simulink model "flockingModel"  (R2018b)
settings: Solver=FixedStepAuto  StartTime=0.0  StopTime=300  FixedStep=0.01  RelTol=1e-3
values from neighbouring files (symbols this model uses):
  a = 0.15    [diff_drive.m]    (also in main.m)
  bias = 0.2    [diff_drive.m]    (also in main.m)
  obsR = 0.15    [main.m]
  theta01 = 0    [main.m]
  theta02 = pi/2    (= 1.57079632679)    [main.m]
  theta03 = pi/4    (= 0.785398163397)    [main.m]
  w = 0.1    [diff_drive.m]    (also in main.m)
  x01 = 0.2    [main.m]
  x02 = 0.07    [main.m]
  x03 = 0.05    [main.m]
  x_obs = 0.20    (= 0.2)    [diff_drive.m]    (also in main.m = 1.5)
  x_star = 0.15    [diff_drive.m]    (also in main.m = 2.2)
  y01 = 0.25    [main.m]
  y02 = 0.5    [main.m]
  y03 = 0.3    [main.m]
  y_obs = 0.2    [diff_drive.m]    (also in main.m = 1)
  y_star = 0.00    (= 0)    [diff_drive.m]    (also in main.m = 1)
settings Model: Creator=root  LastModifiedBy=root

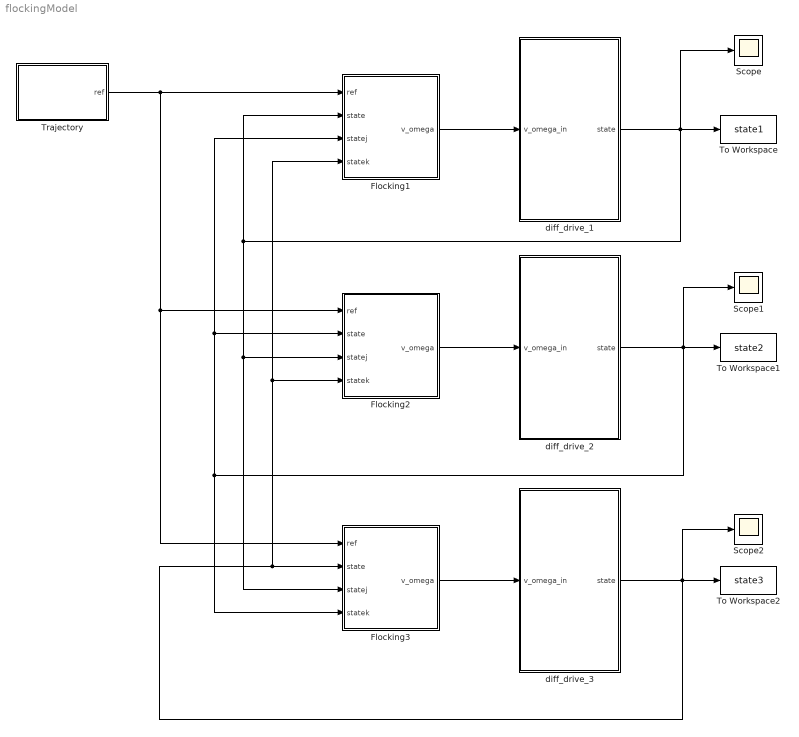
== system flockingModel ==
  Flocking1 : Subsystem
  Flocking2 : Subsystem
  Flocking3 : Subsystem
  Scope : Scope
  Scope1 : Scope
  Scope2 : Scope
  To Workspace : ToWorkspace  VariableName=state1  SaveFormat=Timeseries  SampleTime=-1
  To Workspace1 : ToWorkspace  VariableName=state2  SaveFormat=Timeseries  SampleTime=-1
  To Workspace2 : ToWorkspace  VariableName=state3  SaveFormat=Timeseries  SampleTime=-1
  Trajectory : Subsystem  TreatAsAtomicUnit=on
  diff_drive_1 : Subsystem  mask{base=0.078, base_error=2.5, radius=0.029, radius_error=6.9, omega_max=180}
      mask prompts: base_error "Base error in percent"; radius_error "Radius error in percent"; omega_max "Wheel Max Velocity"
  "diff_drive_2 " : Subsystem  mask{base=0.078, base_error=2.5, radius=0.029, radius_error=6.9, omega_max=180}
      mask prompts: base_error "Base error in percent"; radius_error "Radius error in percent"; omega_max "Wheel Max Velocity"
  diff_drive_3 : Subsystem  mask{base=0.078, base_error=2.5, radius=0.029, radius_error=6.9, omega_max=180}
      mask prompts: base_error "Base error in percent"; radius_error "Radius error in percent"; omega_max "Wheel Max Velocity"
  wires:
  Trajectory/1(ref) -> Flocking1/1(ref), Flocking3/1(ref), Flocking2/1(ref)
  diff_drive_1/1(state) -> Scope/1, To Workspace/1, Flocking1/2(state), Flocking3/3(statej), Flocking2/3(statej)
  Flocking1/1(v_omega) -> diff_drive_1/1(v_omega_in)
  "diff_drive_2 "/1(state) -> Scope1/1, To Workspace1/1, Flocking3/4(statek), Flocking2/2(state), Flocking1/3(statej)
  Flocking2/1(v_omega) -> "diff_drive_2 "/1(v_omega_in)
  Flocking3/1(v_omega) -> diff_drive_3/1(v_omega_in)
  diff_drive_3/1(state) -> Scope2/1, Flocking3/2(state), Flocking2/4(statek), Flocking1/4(statek), To Workspace2/1

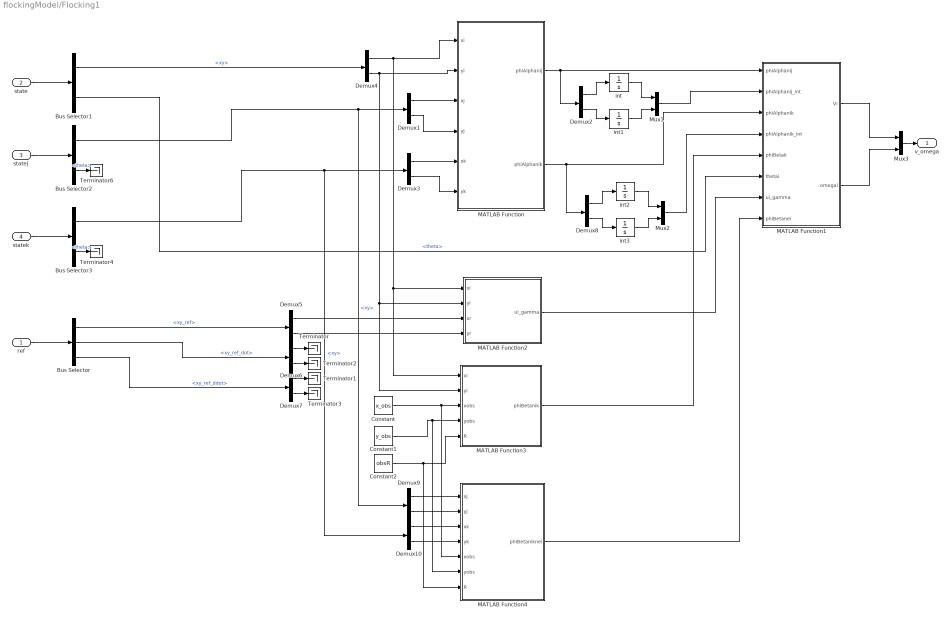
== system flockingModel/Flocking1 ==
  ref : Inport
  state : Inport  Port=2
  statej : Inport  Port=3
  statek : Inport  Port=4
  Bus Selector : BusSelector  OutputSignals=xy_ref,xy_ref_dot,xy_ref_ddot
  Bus Selector1 : BusSelector  OutputSignals=xy,theta
  Bus Selector2 : BusSelector  OutputSignals=xy,theta
  Bus Selector3 : BusSelector  OutputSignals=xy,theta
  Constant : Constant  Value=x_obs
  Constant1 : Constant  Value=y_obs
  Constant2 : Constant  Value=obsR
  Demux{1..10} (10 alike) : Demux  Outputs=2
  MATLAB Function : MATLAB Function  TreatAsAtomicUnit=on
  MATLAB Function1 : MATLAB Function  TreatAsAtomicUnit=on
  MATLAB Function2 : MATLAB Function  TreatAsAtomicUnit=on
  MATLAB Function3 : MATLAB Function  TreatAsAtomicUnit=on
  MATLAB Function4 : MATLAB Function  TreatAsAtomicUnit=on
  Mux1 : Mux  Inputs=2
  Mux2 : Mux  Inputs=2
  Mux3 : Mux  Inputs=2
  Terminator{,1..4,6} (6 alike) : Terminator
  int{,1..3} (4 alike) : Integrator
  v_omega : Outport
  wires:
  ref/1 -> Bus Selector/1
  state/1 -> Bus Selector1/1
  Bus Selector/2 -> Demux6/1  "<xy_ref_dot>"
  Bus Selector/1 -> Demux5/1  "<xy_ref>"
  Bus Selector/3 -> Demux7/1  "<xy_ref_ddot>"
  Bus Selector1/1 -> Demux4/1  "<xy>"
  Mux3/1 -> v_omega/1
  Demux6/1 -> Terminator/1
  Demux6/2 -> Terminator2/1
  Demux7/1 -> Terminator1/1
  Demux7/2 -> Terminator3/1
  statej/1 -> Bus Selector2/1
  Bus Selector2/1 -> Demux9/1, Demux1/1  "<xy>"
  Demux4/1 -> MATLAB Function/1(xi), MATLAB Function3/1(xi), MATLAB Function2/1(xi)
  Demux4/2 -> MATLAB Function/2(yi), MATLAB Function3/2(yi), MATLAB Function2/2(yi)
  Demux1/1 -> MATLAB Function/3(xj)
  Demux1/2 -> MATLAB Function/4(yj)
  MATLAB Function1/1(Vi) -> Mux3/1
  MATLAB Function1/2(omegai) -> Mux3/2
  MATLAB Function/1(phiAlphanij) -> Demux2/1, MATLAB Function1/1(phiAlphanij)
  Demux5/2 -> MATLAB Function2/4(yr)
  Bus Selector2/2 -> Terminator6/1  "<theta>"
  Bus Selector1/2 -> MATLAB Function1/6(thetai)  "<theta>"
  Demux2/1 -> int/1
  Demux2/2 -> int1/1
  int/1 -> Mux1/1
  int1/1 -> Mux1/2
  Mux1/1 -> MATLAB Function1/2(phiAlphanij_int)
  Demux5/1 -> MATLAB Function2/3(xr)
  MATLAB Function2/1(ui_gamma) -> MATLAB Function1/7(ui_gamma)
  statek/1 -> Bus Selector3/1
  Bus Selector3/2 -> Terminator4/1  "<theta>"
  Demux3/1 -> MATLAB Function/5(xk)
  Demux3/2 -> MATLAB Function/6(yk)
  Bus Selector3/1 -> Demux10/1, Demux3/1  "<xy>"
  int3/1 -> Mux2/2
  MATLAB Function/2(phiAlphanik) -> Demux8/1, MATLAB Function1/3(phiAlphanik)
  Demux8/1 -> int2/1
  Demux8/2 -> int3/1
  int2/1 -> Mux2/1
  Mux2/1 -> MATLAB Function1/4(phiAlphanik_int)
  Constant/1 -> MATLAB Function4/5(xobs), MATLAB Function3/3(xobs)
  Constant1/1 -> MATLAB Function4/6(yobs), MATLAB Function3/4(yobs)
  MATLAB Function3/1(phiBetanik) -> MATLAB Function1/5(phiBetak)
  Constant2/1 -> MATLAB Function4/7(R), MATLAB Function3/5(R)
  Demux9/1 -> MATLAB Function4/1(xj)
  Demux9/2 -> MATLAB Function4/2(yj)
  Demux10/1 -> MATLAB Function4/3(xk)
  Demux10/2 -> MATLAB Function4/4(yk)
  MATLAB Function4/1(phiBetaniknei) -> MATLAB Function1/8(phiBetanei)

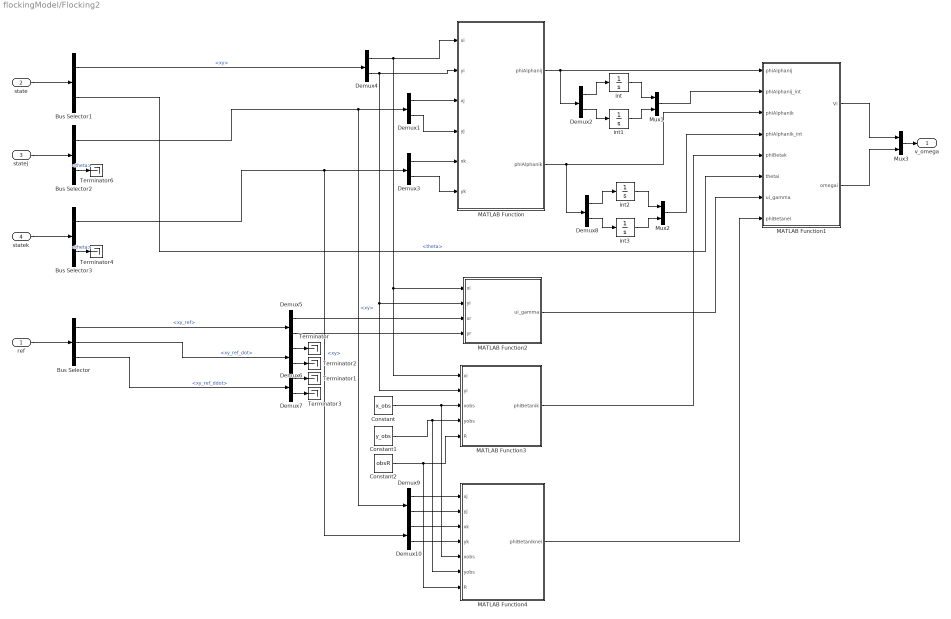
== system flockingModel/Flocking2 ==
  ref : Inport
  state : Inport  Port=2
  statej : Inport  Port=3
  statek : Inport  Port=4
  Bus Selector : BusSelector  OutputSignals=xy_ref,xy_ref_dot,xy_ref_ddot
  Bus Selector1 : BusSelector  OutputSignals=xy,theta
  Bus Selector2 : BusSelector  OutputSignals=xy,theta
  Bus Selector3 : BusSelector  OutputSignals=xy,theta
  Constant : Constant  Value=x_obs
  Constant1 : Constant  Value=y_obs
  Constant2 : Constant  Value=obsR
  Demux{1..10} (10 alike) : Demux  Outputs=2
  MATLAB Function : MATLAB Function  TreatAsAtomicUnit=on
  MATLAB Function1 : MATLAB Function  TreatAsAtomicUnit=on
  MATLAB Function2 : MATLAB Function  TreatAsAtomicUnit=on
  MATLAB Function3 : MATLAB Function  TreatAsAtomicUnit=on
  MATLAB Function4 : MATLAB Function  TreatAsAtomicUnit=on
  Mux1 : Mux  Inputs=2
  Mux2 : Mux  Inputs=2
  Mux3 : Mux  Inputs=2
  Terminator{,1..4,6} (6 alike) : Terminator
  int{,1..3} (4 alike) : Integrator
  v_omega : Outport
  wires:
  ref/1 -> Bus Selector/1
  state/1 -> Bus Selector1/1
  Bus Selector/2 -> Demux6/1  "<xy_ref_dot>"
  Bus Selector/1 -> Demux5/1  "<xy_ref>"
  Bus Selector/3 -> Demux7/1  "<xy_ref_ddot>"
  Bus Selector1/1 -> Demux4/1  "<xy>"
  Mux3/1 -> v_omega/1
  Demux6/1 -> Terminator/1
  Demux6/2 -> Terminator2/1
  Demux7/1 -> Terminator1/1
  Demux7/2 -> Terminator3/1
  statej/1 -> Bus Selector2/1
  Bus Selector2/1 -> Demux9/1, Demux1/1  "<xy>"
  Demux4/1 -> MATLAB Function/1(xi), MATLAB Function3/1(xi), MATLAB Function2/1(xi)
  Demux4/2 -> MATLAB Function/2(yi), MATLAB Function3/2(yi), MATLAB Function2/2(yi)
  Demux1/1 -> MATLAB Function/3(xj)
  Demux1/2 -> MATLAB Function/4(yj)
  MATLAB Function1/1(Vi) -> Mux3/1
  MATLAB Function1/2(omegai) -> Mux3/2
  MATLAB Function/1(phiAlphanij) -> Demux2/1, MATLAB Function1/1(phiAlphanij)
  Demux5/2 -> MATLAB Function2/4(yr)
  Bus Selector2/2 -> Terminator6/1  "<theta>"
  Bus Selector1/2 -> MATLAB Function1/6(thetai)  "<theta>"
  Demux2/1 -> int/1
  Demux2/2 -> int1/1
  int/1 -> Mux1/1
  int1/1 -> Mux1/2
  Mux1/1 -> MATLAB Function1/2(phiAlphanij_int)
  Demux5/1 -> MATLAB Function2/3(xr)
  MATLAB Function2/1(ui_gamma) -> MATLAB Function1/7(ui_gamma)
  statek/1 -> Bus Selector3/1
  Bus Selector3/2 -> Terminator4/1  "<theta>"
  Demux3/1 -> MATLAB Function/5(xk)
  Demux3/2 -> MATLAB Function/6(yk)
  Bus Selector3/1 -> Demux10/1, Demux3/1  "<xy>"
  int3/1 -> Mux2/2
  MATLAB Function/2(phiAlphanik) -> Demux8/1, MATLAB Function1/3(phiAlphanik)
  Demux8/1 -> int2/1
  Demux8/2 -> int3/1
  int2/1 -> Mux2/1
  Mux2/1 -> MATLAB Function1/4(phiAlphanik_int)
  Constant/1 -> MATLAB Function4/5(xobs), MATLAB Function3/3(xobs)
  Constant1/1 -> MATLAB Function4/6(yobs), MATLAB Function3/4(yobs)
  MATLAB Function3/1(phiBetanik) -> MATLAB Function1/5(phiBetak)
  Constant2/1 -> MATLAB Function4/7(R), MATLAB Function3/5(R)
  Demux9/1 -> MATLAB Function4/1(xj)
  Demux9/2 -> MATLAB Function4/2(yj)
  Demux10/1 -> MATLAB Function4/3(xk)
  Demux10/2 -> MATLAB Function4/4(yk)
  MATLAB Function4/1(phiBetaniknei) -> MATLAB Function1/8(phiBetanei)

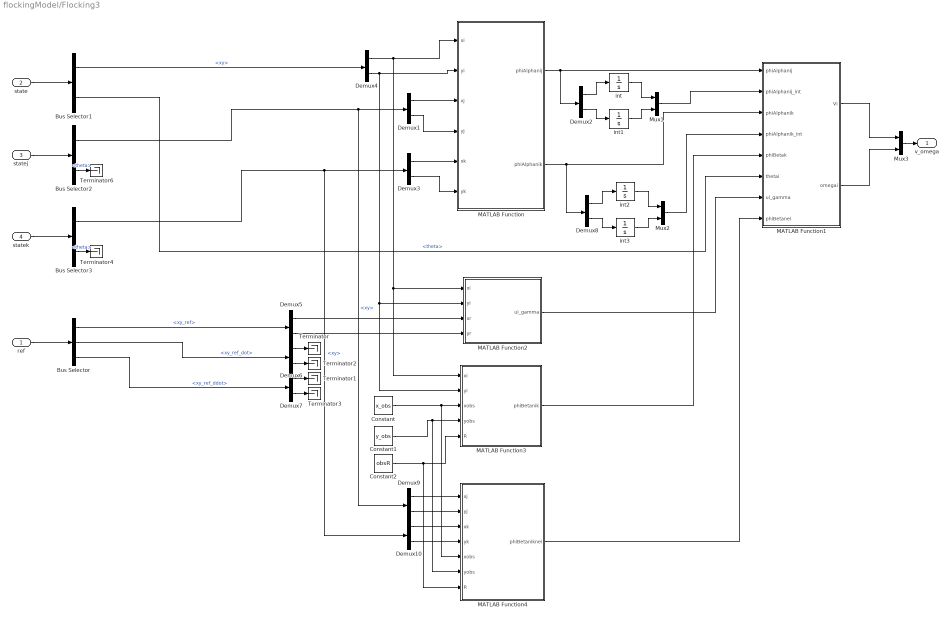
== system flockingModel/Flocking3 ==
  ref : Inport
  state : Inport  Port=2
  statej : Inport  Port=3
  statek : Inport  Port=4
  Bus Selector : BusSelector  OutputSignals=xy_ref,xy_ref_dot,xy_ref_ddot
  Bus Selector1 : BusSelector  OutputSignals=xy,theta
  Bus Selector2 : BusSelector  OutputSignals=xy,theta
  Bus Selector3 : BusSelector  OutputSignals=xy,theta
  Constant : Constant  Value=x_obs
  Constant1 : Constant  Value=y_obs
  Constant2 : Constant  Value=obsR
  Demux{1..10} (10 alike) : Demux  Outputs=2
  MATLAB Function : MATLAB Function  TreatAsAtomicUnit=on
  MATLAB Function1 : MATLAB Function  TreatAsAtomicUnit=on
  MATLAB Function2 : MATLAB Function  TreatAsAtomicUnit=on
  MATLAB Function3 : MATLAB Function  TreatAsAtomicUnit=on
  MATLAB Function4 : MATLAB Function  TreatAsAtomicUnit=on
  Mux1 : Mux  Inputs=2
  Mux2 : Mux  Inputs=2
  Mux3 : Mux  Inputs=2
  Terminator{,1..4,6} (6 alike) : Terminator
  int{,1..3} (4 alike) : Integrator
  v_omega : Outport
  wires:
  ref/1 -> Bus Selector/1
  state/1 -> Bus Selector1/1
  Bus Selector/2 -> Demux6/1  "<xy_ref_dot>"
  Bus Selector/1 -> Demux5/1  "<xy_ref>"
  Bus Selector/3 -> Demux7/1  "<xy_ref_ddot>"
  Bus Selector1/1 -> Demux4/1  "<xy>"
  Mux3/1 -> v_omega/1
  Demux6/1 -> Terminator/1
  Demux6/2 -> Terminator2/1
  Demux7/1 -> Terminator1/1
  Demux7/2 -> Terminator3/1
  statej/1 -> Bus Selector2/1
  Bus Selector2/1 -> Demux9/1, Demux1/1  "<xy>"
  Demux4/1 -> MATLAB Function/1(xi), MATLAB Function3/1(xi), MATLAB Function2/1(xi)
  Demux4/2 -> MATLAB Function/2(yi), MATLAB Function3/2(yi), MATLAB Function2/2(yi)
  Demux1/1 -> MATLAB Function/3(xj)
  Demux1/2 -> MATLAB Function/4(yj)
  MATLAB Function1/1(Vi) -> Mux3/1
  MATLAB Function1/2(omegai) -> Mux3/2
  MATLAB Function/1(phiAlphanij) -> Demux2/1, MATLAB Function1/1(phiAlphanij)
  Demux5/2 -> MATLAB Function2/4(yr)
  Bus Selector2/2 -> Terminator6/1  "<theta>"
  Bus Selector1/2 -> MATLAB Function1/6(thetai)  "<theta>"
  Demux2/1 -> int/1
  Demux2/2 -> int1/1
  int/1 -> Mux1/1
  int1/1 -> Mux1/2
  Mux1/1 -> MATLAB Function1/2(phiAlphanij_int)
  Demux5/1 -> MATLAB Function2/3(xr)
  MATLAB Function2/1(ui_gamma) -> MATLAB Function1/7(ui_gamma)
  statek/1 -> Bus Selector3/1
  Bus Selector3/2 -> Terminator4/1  "<theta>"
  Demux3/1 -> MATLAB Function/5(xk)
  Demux3/2 -> MATLAB Function/6(yk)
  Bus Selector3/1 -> Demux10/1, Demux3/1  "<xy>"
  int3/1 -> Mux2/2
  MATLAB Function/2(phiAlphanik) -> Demux8/1, MATLAB Function1/3(phiAlphanik)
  Demux8/1 -> int2/1
  Demux8/2 -> int3/1
  int2/1 -> Mux2/1
  Mux2/1 -> MATLAB Function1/4(phiAlphanik_int)
  Constant/1 -> MATLAB Function4/5(xobs), MATLAB Function3/3(xobs)
  Constant1/1 -> MATLAB Function4/6(yobs), MATLAB Function3/4(yobs)
  MATLAB Function3/1(phiBetanik) -> MATLAB Function1/5(phiBetak)
  Constant2/1 -> MATLAB Function4/7(R), MATLAB Function3/5(R)
  Demux9/1 -> MATLAB Function4/1(xj)
  Demux9/2 -> MATLAB Function4/2(yj)
  Demux10/1 -> MATLAB Function4/3(xk)
  Demux10/2 -> MATLAB Function4/4(yk)
  MATLAB Function4/1(phiBetaniknei) -> MATLAB Function1/8(phiBetanei)

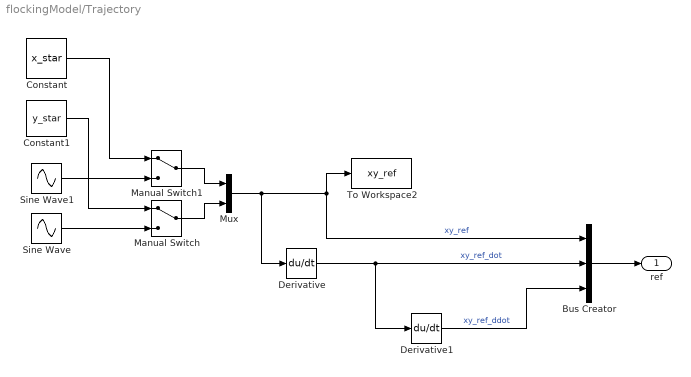
== system flockingModel/Trajectory ==
  Bus Creator : BusCreator  Inputs=3
  Constant : Constant  Value=x_star
  Constant1 : Constant  Value=y_star
  Derivative : Derivative
  Derivative1 : Derivative
  Manual Switch : ManualSwitch
  Manual Switch1 : ManualSwitch
  Mux : Mux  Inputs=2
  Sine Wave : Sin  Amplitude=a  Bias=bias  Frequency=w  SampleTime=0
  Sine Wave1 : Sin  Amplitude=a  Bias=bias  Frequency=w  Phase=pi/2  SampleTime=0
  To Workspace2 : ToWorkspace  VariableName=xy_ref  SampleTime=-1
      settings: Save2DSignal=2-D array (concatenate along first dimension)
  ref : Outport
  wires:
  Bus Creator/1 -> ref/1
  Mux/1 -> Derivative/1, Bus Creator/1, To Workspace2/1  "xy_ref"
  Derivative/1 -> Bus Creator/2, Derivative1/1  "xy_ref_dot"
  Derivative1/1 -> Bus Creator/3  "xy_ref_ddot"
  Sine Wave/1 -> Manual Switch/2
  Sine Wave1/1 -> Manual Switch1/2
  Constant/1 -> Manual Switch1/1
  Constant1/1 -> Manual Switch/1
  Manual Switch1/1 -> Mux/1
  Manual Switch/1 -> Mux/2

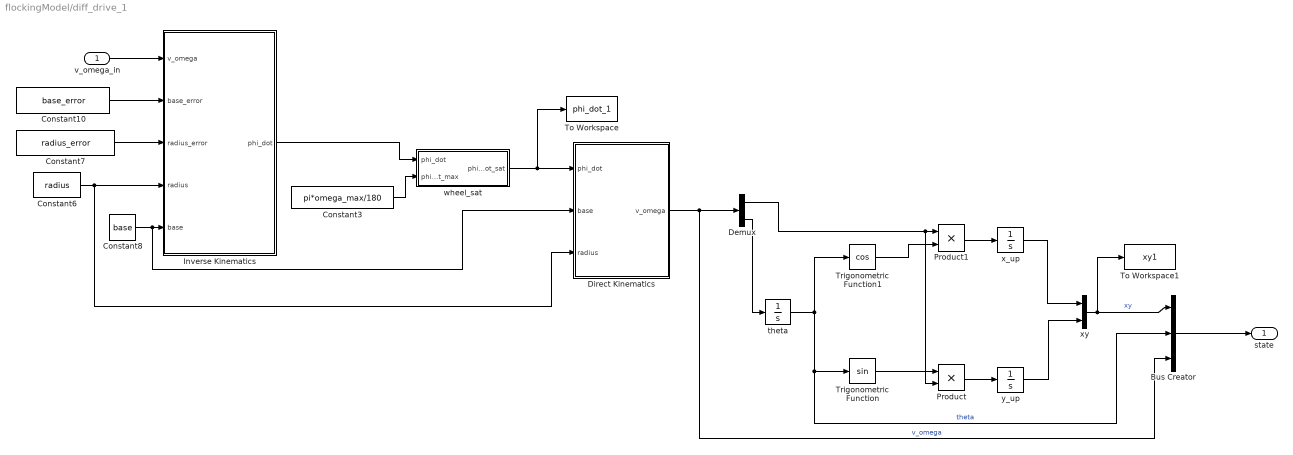
== system flockingModel/diff_drive_1 ==
  v_omega_in : Inport
  Bus Creator : BusCreator  Inputs=3
  Constant10 : Constant  Value=base_error
  Constant3 : Constant  Value=pi*omega_max/180
  Constant6 : Constant  Value=radius
  Constant7 : Constant  Value=radius_error
  Constant8 : Constant  Value=base
  Demux : Demux  Outputs=2
  Direct Kinematics : MATLAB Function  TreatAsAtomicUnit=on
  Inverse Kinematics : MATLAB Function  TreatAsAtomicUnit=on
  Product : Product
  Product1 : Product
  To Workspace : ToWorkspace  VariableName=phi_dot_1  SampleTime=-1
      settings: Save2DSignal=2-D array (concatenate along first dimension)
  To Workspace1 : ToWorkspace  VariableName=xy1  SampleTime=-1
      settings: Save2DSignal=2-D array (concatenate along first dimension)
  Trigonometric Function : Trigonometry
  Trigonometric Function1 : Trigonometry  Operator=cos
  theta : Integrator  InitialCondition=theta01
  wheel_sat : Subsystem
  x_up : Integrator  InitialCondition=x01
  xy : Mux  Inputs=2
  y_up : Integrator  InitialCondition=y01
  state : Outport
  wires:
  theta/1 -> Trigonometric Function1/1, Trigonometric Function/1, Bus Creator/2  "theta"
  Trigonometric Function1/1 -> Product1/2
  Trigonometric Function/1 -> Product/1
  Product/1 -> y_up/1
  Product1/1 -> x_up/1
  x_up/1 -> xy/1
  Constant3/1 -> wheel_sat/2(phi_dot_max)
  Direct Kinematics/1(v_omega) -> Bus Creator/3, Demux/1  "v_omega"
  Demux/1 -> Product/2, Product1/1
  Demux/2 -> theta/1
  y_up/1 -> xy/2
  wheel_sat/1(phi_dot_sat) -> Direct Kinematics/1(phi_dot), To Workspace/1
  xy/1 -> Bus Creator/1, To Workspace1/1  "xy"
  Bus Creator/1 -> state/1
  Inverse Kinematics/1(phi_dot) -> wheel_sat/1(phi_dot)
  v_omega_in/1 -> Inverse Kinematics/1(v_omega)
  Constant10/1 -> Inverse Kinematics/2(base_error)
  Constant7/1 -> Inverse Kinematics/3(radius_error)
  Constant6/1 -> Inverse Kinematics/4(radius), Direct Kinematics/3(radius)
  Constant8/1 -> Direct Kinematics/2(base), Inverse Kinematics/5(base)

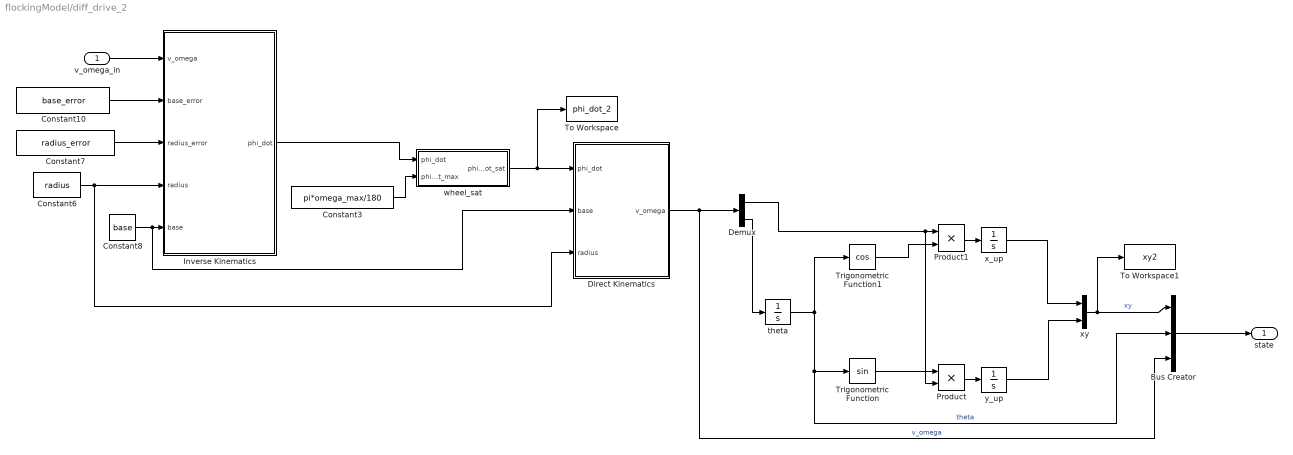
== system flockingModel/diff_drive_2  ==
  v_omega_in : Inport
  Bus Creator : BusCreator  Inputs=3
  Constant10 : Constant  Value=base_error
  Constant3 : Constant  Value=pi*omega_max/180
  Constant6 : Constant  Value=radius
  Constant7 : Constant  Value=radius_error
  Constant8 : Constant  Value=base
  Demux : Demux  Outputs=2
  Direct Kinematics : MATLAB Function  TreatAsAtomicUnit=on
  Inverse Kinematics : MATLAB Function  TreatAsAtomicUnit=on
  Product : Product
  Product1 : Product
  To Workspace : ToWorkspace  VariableName=phi_dot_2  SampleTime=-1
      settings: Save2DSignal=2-D array (concatenate along first dimension)
  To Workspace1 : ToWorkspace  VariableName=xy2  SampleTime=-1
      settings: Save2DSignal=2-D array (concatenate along first dimension)
  Trigonometric Function : Trigonometry
  Trigonometric Function1 : Trigonometry  Operator=cos
  theta : Integrator  InitialCondition=theta02
  wheel_sat : Subsystem
  x_up : Integrator  InitialCondition=x02
  xy : Mux  Inputs=2
  y_up : Integrator  InitialCondition=y02
  state : Outport
  wires:
  Constant8/1 -> Inverse Kinematics/5(base), Direct Kinematics/2(base)
  Constant6/1 -> Direct Kinematics/3(radius), Inverse Kinematics/4(radius)
  Constant7/1 -> Inverse Kinematics/3(radius_error)
  Constant10/1 -> Inverse Kinematics/2(base_error)
  v_omega_in/1 -> Inverse Kinematics/1(v_omega)
  Inverse Kinematics/1(phi_dot) -> wheel_sat/1(phi_dot)
  Bus Creator/1 -> state/1
  xy/1 -> To Workspace1/1, Bus Creator/1  "xy"
  wheel_sat/1(phi_dot_sat) -> To Workspace/1, Direct Kinematics/1(phi_dot)
  y_up/1 -> xy/2
  Demux/2 -> theta/1
  Demux/1 -> Product1/1, Product/2
  Direct Kinematics/1(v_omega) -> Demux/1, Bus Creator/3  "v_omega"
  Constant3/1 -> wheel_sat/2(phi_dot_max)
  x_up/1 -> xy/1
  Product1/1 -> x_up/1
  Product/1 -> y_up/1
  Trigonometric Function/1 -> Product/1
  Trigonometric Function1/1 -> Product1/2
  theta/1 -> Bus Creator/2, Trigonometric Function/1, Trigonometric Function1/1  "theta"

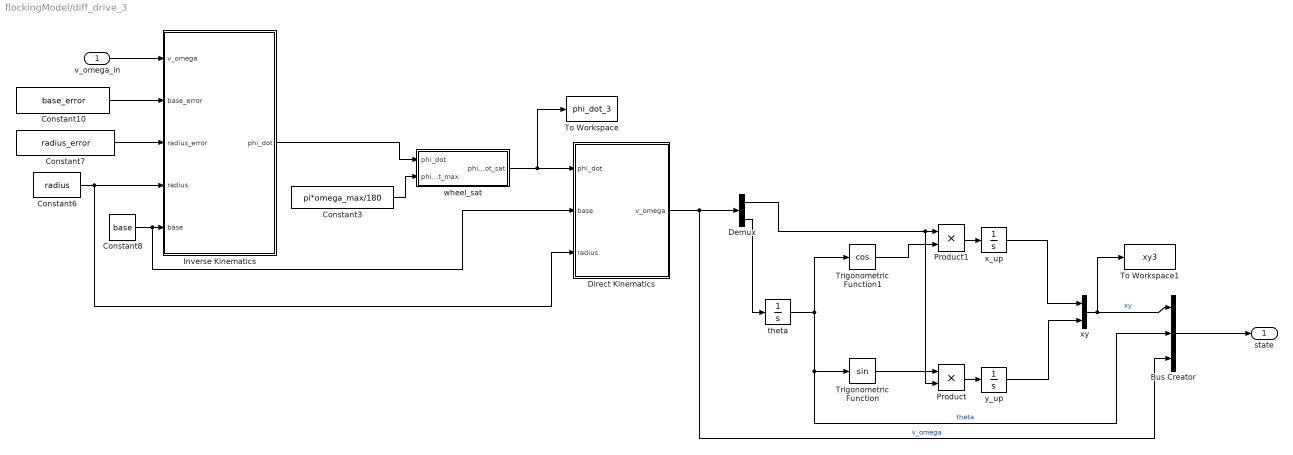
== system flockingModel/diff_drive_3 ==
  v_omega_in : Inport
  Bus Creator : BusCreator  Inputs=3
  Constant10 : Constant  Value=base_error
  Constant3 : Constant  Value=pi*omega_max/180
  Constant6 : Constant  Value=radius
  Constant7 : Constant  Value=radius_error
  Constant8 : Constant  Value=base
  Demux : Demux  Outputs=2
  Direct Kinematics : MATLAB Function  TreatAsAtomicUnit=on
  Inverse Kinematics : MATLAB Function  TreatAsAtomicUnit=on
  Product : Product
  Product1 : Product
  To Workspace : ToWorkspace  VariableName=phi_dot_3  SampleTime=-1
      settings: Save2DSignal=2-D array (concatenate along first dimension)
  To Workspace1 : ToWorkspace  VariableName=xy3  SampleTime=-1
      settings: Save2DSignal=2-D array (concatenate along first dimension)
  Trigonometric Function : Trigonometry
  Trigonometric Function1 : Trigonometry  Operator=cos
  theta : Integrator  InitialCondition=theta03
  wheel_sat : Subsystem
  x_up : Integrator  InitialCondition=x03
  xy : Mux  Inputs=2
  y_up : Integrator  InitialCondition=y03
  state : Outport
  wires:
  Constant8/1 -> Inverse Kinematics/5(base), Direct Kinematics/2(base)
  Constant6/1 -> Direct Kinematics/3(radius), Inverse Kinematics/4(radius)
  Constant7/1 -> Inverse Kinematics/3(radius_error)
  Constant10/1 -> Inverse Kinematics/2(base_error)
  v_omega_in/1 -> Inverse Kinematics/1(v_omega)
  Inverse Kinematics/1(phi_dot) -> wheel_sat/1(phi_dot)
  Bus Creator/1 -> state/1
  xy/1 -> To Workspace1/1, Bus Creator/1  "xy"
  wheel_sat/1(phi_dot_sat) -> To Workspace/1, Direct Kinematics/1(phi_dot)
  y_up/1 -> xy/2
  Demux/2 -> theta/1
  Demux/1 -> Product1/1, Product/2
  Direct Kinematics/1(v_omega) -> Demux/1, Bus Creator/3  "v_omega"
  Constant3/1 -> wheel_sat/2(phi_dot_max)
  x_up/1 -> xy/1
  Product1/1 -> x_up/1
  Product/1 -> y_up/1
  Trigonometric Function/1 -> Product/1
  Trigonometric Function1/1 -> Product1/2
  theta/1 -> Bus Creator/2, Trigonometric Function/1, Trigonometric Function1/1  "theta"

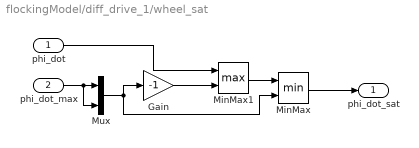
== system flockingModel/diff_drive_1/wheel_sat ==
  phi_dot : Inport
  phi_dot_max : Inport  Port=2
  Gain : Gain  Gain=-1
  MinMax : MinMax  Inputs=2
  MinMax1 : MinMax  Function=max  Inputs=2
  Mux : Mux  Inputs=2
  phi_dot_sat : Outport
  wires:
  Gain/1 -> MinMax1/2
  MinMax/1 -> phi_dot_sat/1
  phi_dot_max/1 -> Mux/2, Mux/1
  phi_dot/1 -> MinMax1/1
  MinMax1/1 -> MinMax/1
  Mux/1 -> MinMax/2, Gain/1

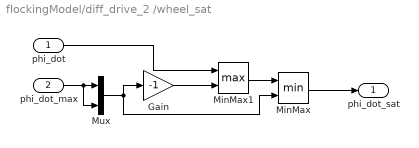
== system flockingModel/diff_drive_2 /wheel_sat ==
  phi_dot : Inport
  phi_dot_max : Inport  Port=2
  Gain : Gain  Gain=-1
  MinMax : MinMax  Inputs=2
  MinMax1 : MinMax  Function=max  Inputs=2
  Mux : Mux  Inputs=2
  phi_dot_sat : Outport
  wires:
  Mux/1 -> Gain/1, MinMax/2
  MinMax1/1 -> MinMax/1
  phi_dot/1 -> MinMax1/1
  phi_dot_max/1 -> Mux/1, Mux/2
  MinMax/1 -> phi_dot_sat/1
  Gain/1 -> MinMax1/2

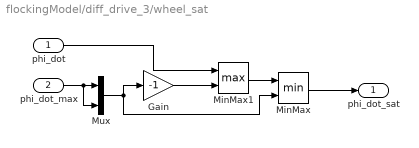
== system flockingModel/diff_drive_3/wheel_sat ==
  phi_dot : Inport
  phi_dot_max : Inport  Port=2
  Gain : Gain  Gain=-1
  MinMax : MinMax  Inputs=2
  MinMax1 : MinMax  Function=max  Inputs=2
  Mux : Mux  Inputs=2
  phi_dot_sat : Outport
  wires:
  Mux/1 -> Gain/1, MinMax/2
  MinMax1/1 -> MinMax/1
  phi_dot/1 -> MinMax1/1
  phi_dot_max/1 -> Mux/1, Mux/2
  MinMax/1 -> phi_dot_sat/1
  Gain/1 -> MinMax1/2

== matlab function flockingModel/diff_drive_1/Inverse Kinematics ==
  data: v_omega input; base_error input; radius_error input; radius input; phi_dot output; base input
function phi_dot = ik(v_omega, base_error, radius_error, radius, base)

base = base * (1+base_error*0.01);
radius = radius * (1+radius_error*0.01);

phi_dot = [(v_omega(1)+base*v_omega(2))/radius; (v_omega(1)-base*v_omega(2))/radius];

== matlab function flockingModel/Flocking1/MATLAB Function1 ==
  data: phiAlphanij input; phiAlphanij_int input; phiAlphanik input; phiAlphanik_int input; phiBetak input; thetai input; Vi output; omegai output; ui_gamma input; phiBetanei input

function [Vi, omegai]  = ctrlLaw(phiAlphanij, phiAlphanij_int, phiAlphanik, phiAlphanik_int, phiBetak, thetai, ui_gamma, phiBetanei)
    
    % Control gains and parameters
    Kp = 4.5 ;%4.5 ; %5.50 ; % 7.5
    Ki = 0.45 ; %0.35 ; % 0.05
    l = 0.01 ;
    
    cBeta = 0.2; % 0.2
    
    Ktheta = [cos(thetai), sin(thetai) ;
              -sin(thetai)/l, cos(thetai)/l ] ;
    
    hx_dot = Kp * phiAlphanij(1,1) + Ki * phiAlphanij_int(1,1) + Kp * phiAlphanik(1,1) + Ki * phiAlphanik_int(1,1) + cBeta * (phiBetak(1,1) + phiBetanei(1,1)) + ui_gamma(1,1) ;
    hy_dot = Kp * phiAlphanij(2,1) + Ki * phiAlphanij_int(2,1) + Kp * phiAlphanik(2,1) + Ki * phiAlphanik_int(2,1) + cBeta * (phiBetak(2,1) + phiBetanei(2,1)) + ui_gamma(2,1) ;
    
    %hx_dot = Kp * phiAlphanij(1,1) + Ki * phiAlphanij_int(1,1) + Kp * phiAlphanik(1,1) + Ki * phiAlphanik_int(1,1) + cBeta * (phiBetak(1,1)) + ui_gamma(1,1) ;
    %hy_dot = Kp * phiAlphanij(2,1) + Ki * phiAlphanij_int(2,1) + Kp * phiAlphanik(2,1) + Ki * phiAlphanik_int(2,1) + cBeta * (phiBetak(2,1)) + ui_gamma(2,1) ;
    
    Ui = Ktheta * [hx_dot ; hy_dot] ;
    Vi = Ui(1,1) ;
    omegai = Ui(2,1) ;
    
end

== matlab function flockingModel/Flocking1/MATLAB Function ==
  data: xi input; yi input; phiAlphanij output; xj input; yj input; xk input; yk input; phiAlphanik output

function [phiAlphanij, phiAlphanik]  = phiAlphaFcn(xi, yi, xj, yj, xk, yk)
    
    % Parameters
    epsilon = 0.1 ;
    a = 1 ;        % 0 < a <= b
    b = 1 ;
    c = 0.6 ;     % 0.6 
    d = 0.3 ;     % 0.3
    e = abs(a - b) / sqrt(4*a*b) ;
    h = 0.2 ;
    cAlpha = sigmaNormFun(c, epsilon) ;
    dAlpha = sigmaNormFun(d, epsilon) ;
    
    Pi = [xi ; yi] ;
    Pj = [xj ; yj] ;
    Pk = [xk ; yk] ;
    
    sigmaNormj = sigmaNormFun(Pj - Pi, epsilon) ;
    nij = gradSigmaFun(Pj - Pi, epsilon) ;
    
    sigmaNormk = sigmaNormFun(Pk - Pi, epsilon) ;
    nik = gradSigmaFun(Pk - Pi, epsilon) ;
    
    sigma1j = sigma1Fun(sigmaNormj - dAlpha + e) ;
    sigma1k = sigma1Fun(sigmaNormk - dAlpha + e) ;
    
    phiAlphaj = 0.5 * bumpFcn(sigmaNormj/cAlpha,h) * ((a+b)*sigma1j + (a-b)) ;
    phiAlphanij = phiAlphaj.* nij ;
    
    phiAlphak = 0.5 * bumpFcn(sigmaNormk/cAlpha,h) * ((a+b)*sigma1k + (a-b)) ;
    phiAlphanik = phiAlphak.* nik ;
    
end

== matlab function flockingModel/diff_drive_1/Direct Kinematics ==
  data: phi_dot input; v_omega output; base input; radius input
function v_omega = dk(phi_dot, base, radius)

v_omega = [radius*(phi_dot(1)+phi_dot(2))/2; radius*(phi_dot(1)-phi_dot(2))/(2*base)];

== matlab function flockingModel/Flocking2/MATLAB Function ==
  data: xi input; yi input; phiAlphanij output; xj input; yj input; xk input; yk input; phiAlphanik output

function [phiAlphanij, phiAlphanik]  = phiAlphaFcn(xi, yi, xj, yj, xk, yk)
    
    % Parameters
    epsilon = 0.1 ;
    a = 1 ;        % 0 < a <= b
    b = 1 ;
    c = 0.6 ;     % 0.6 
    d = 0.3 ;     % 0.3
    e = abs(a - b) / sqrt(4*a*b) ;
    h = 0.2 ;
    cAlpha = sigmaNormFun(c, epsilon) ;
    dAlpha = sigmaNormFun(d, epsilon) ;
    
    Pi = [xi ; yi] ;
    Pj = [xj ; yj] ;
    Pk = [xk ; yk] ;
    
    sigmaNormj = sigmaNormFun(Pj - Pi, epsilon) ;
    nij = gradSigmaFun(Pj - Pi, epsilon) ;
    
    sigmaNormk = sigmaNormFun(Pk - Pi, epsilon) ;
    nik = gradSigmaFun(Pk - Pi, epsilon) ;
    
    sigma1j = sigma1Fun(sigmaNormj - dAlpha + e) ;
    sigma1k = sigma1Fun(sigmaNormk - dAlpha + e) ;
    
    phiAlphaj = 0.5 * bumpFcn(sigmaNormj/cAlpha,h) * ((a+b)*sigma1j + (a-b)) ;
    phiAlphanij = phiAlphaj.* nij ;
    
    phiAlphak = 0.5 * bumpFcn(sigmaNormk/cAlpha,h) * ((a+b)*sigma1k + (a-b)) ;
    phiAlphanik = phiAlphak.* nik ;
    
end

== matlab function flockingModel/Flocking2/MATLAB Function1 ==
  data: phiAlphanij input; phiAlphanij_int input; phiAlphanik input; phiAlphanik_int input; phiBetak input; thetai input; Vi output; omegai output; ui_gamma input; phiBetanei input

function [Vi, omegai]  = ctrlLaw(phiAlphanij, phiAlphanij_int, phiAlphanik, phiAlphanik_int, phiBetak, thetai, ui_gamma, phiBetanei)
    
    % Control gains and parameters
    Kp = 4.5 ;%4.5 ; %5.50 ; % 7.5
    Ki = 0.45 ; %0.35 ; % 0.05
    l = 0.01 ;
    
    cBeta = 0.2; % 0.2
    
    Ktheta = [cos(thetai), sin(thetai) ;
              -sin(thetai)/l, cos(thetai)/l ] ;
    
    hx_dot = Kp * phiAlphanij(1,1) + Ki * phiAlphanij_int(1,1) + Kp * phiAlphanik(1,1) + Ki * phiAlphanik_int(1,1) + cBeta * (phiBetak(1,1) + phiBetanei(1,1)) + ui_gamma(1,1) ;
    hy_dot = Kp * phiAlphanij(2,1) + Ki * phiAlphanij_int(2,1) + Kp * phiAlphanik(2,1) + Ki * phiAlphanik_int(2,1) + cBeta * (phiBetak(2,1) + phiBetanei(2,1)) + ui_gamma(2,1) ;
    
    %hx_dot = Kp * phiAlphanij(1,1) + Ki * phiAlphanij_int(1,1) + Kp * phiAlphanik(1,1) + Ki * phiAlphanik_int(1,1) + cBeta * (phiBetak(1,1)) + ui_gamma(1,1) ;
    %hy_dot = Kp * phiAlphanij(2,1) + Ki * phiAlphanij_int(2,1) + Kp * phiAlphanik(2,1) + Ki * phiAlphanik_int(2,1) + cBeta * (phiBetak(2,1)) + ui_gamma(2,1) ;
    
    Ui = Ktheta * [hx_dot ; hy_dot] ;
    Vi = Ui(1,1) ;
    omegai = Ui(2,1) ;
    
end

== matlab function flockingModel/diff_drive_2 /Direct Kinematics ==
  data: phi_dot input; v_omega output; base input; radius input
function v_omega = dk(phi_dot, base, radius)

v_omega = [radius*(phi_dot(1)+phi_dot(2))/2; radius*(phi_dot(1)-phi_dot(2))/(2*base)];

== matlab function flockingModel/diff_drive_2 /Inverse Kinematics ==
  data: v_omega input; base_error input; radius_error input; radius input; phi_dot output; base input
function phi_dot = ik(v_omega, base_error, radius_error, radius, base)

base = base * (1+base_error*0.01);
radius = radius * (1+radius_error*0.01);

phi_dot = [(v_omega(1)+base*v_omega(2))/radius; (v_omega(1)-base*v_omega(2))/radius];

== matlab function flockingModel/Flocking1/MATLAB Function2 ==
  data: xi input; yi input; ui_gamma output; xr input; yr input

function ui_gamma   = naviFeedback(xi, yi, xr, yr)
    
    % Control gains
    c_gamma = 0.04 ;
    xmin = -0.03 ;
    xmax = 0.03 ;
    
    Pi = [xi ; yi ] ;
    Pr = [xr ; yr ] ;
    
    ui_gamma = (-1).* satFcn(c_gamma.*(Pi - Pr), xmin, xmax) ;
    
    %Vi_gamma =  - ui_gamma(1,1) ;
    %omegai_gamma = - ui_gamma(2,1) ;
    
end

== matlab function flockingModel/Flocking2/MATLAB Function2 ==
  data: xi input; yi input; ui_gamma output; xr input; yr input

function ui_gamma   = naviFeedback(xi, yi, xr, yr)
    
    % Control gains
    c_gamma = 0.04 ;
    xmin = -0.03 ;
    xmax = 0.03 ;
    
    Pi = [xi ; yi ] ;
    Pr = [xr ; yr ] ;
    
    ui_gamma = (-1).* satFcn(c_gamma.*(Pi - Pr), xmin, xmax) ;
    
    %Vi_gamma =  - ui_gamma(1,1) ;
    %omegai_gamma = - ui_gamma(2,1) ;
    
end

== matlab function flockingModel/diff_drive_3/Direct Kinematics ==
  data: phi_dot input; v_omega output; base input; radius input
function v_omega = dk(phi_dot, base, radius)

v_omega = [radius*(phi_dot(1)+phi_dot(2))/2; radius*(phi_dot(1)-phi_dot(2))/(2*base)];

== matlab function flockingModel/diff_drive_3/Inverse Kinematics ==
  data: v_omega input; base_error input; radius_error input; radius input; phi_dot output; base input
function phi_dot = ik(v_omega, base_error, radius_error, radius, base)

base = base * (1+base_error*0.01);
radius = radius * (1+radius_error*0.01);

phi_dot = [(v_omega(1)+base*v_omega(2))/radius; (v_omega(1)-base*v_omega(2))/radius];

== matlab function flockingModel/Flocking2/MATLAB Function3 ==
  data: xi input; yi input; phiBetanik output; xobs input; yobs input; R input
function phiBetanik = phiBetaFcn(xi, yi, xobs, yobs, R)
    
    % Parameters
    epsilon = 0.1 ;
%     a = 1 ;        % 0 < a <= b
%     b = 1 ;
%     c_prime = 1 ;     % 60cm
    d_prime = 0.37 ;     % 25cm
%     e = abs(a - b) / sqrt(4*a*b) ;
    h = 0.2 ;           % 0.2
%     cBeta = sigmaNormFun(c_prime, epsilon) ;
    dBeta = sigmaNormFun(d_prime, epsilon) ;
    
    Pi = [xi ; yi] ;
    Pc = [xobs ; yobs] ;
    % Compute closest point between the robot center and the obstacle
    % circumference (ossumming obstacles are circles)
    Pk = Pc + (Pi - Pc) * (R /norm(Pi - Pc)) ;
    %Pk = [xobs ; yobs] ;
    
    sigmaNormk = sigmaNormFun(Pk - Pi, epsilon) ;
    nik = gradSigmaFun(Pk - Pi, epsilon) ;
    
    sigma1k = sigma1Fun(sigmaNormk - dBeta) ;
    
    phiBetak = bumpFcn(sigmaNormk/dBeta,h) * (sigma1k - 1) ;
    phiBetanik = phiBetak.* nik ;
    
end

== matlab function flockingModel/Flocking2/MATLAB Function4 ==
  data: xj input; yj input; xk input; yk input; phiBetaniknei output; xobs input; yobs input; R input
function phiBetaniknei = phiBetaFcn(xj, yj, xk, yk, xobs, yobs, R)
    
    % Parameters
    epsilon = 0.1 ;
%     a = 1 ;        % 0 < a <= b
%     b = 1 ;
%     c_prime = 1 ;     % 60cm
    d_prime = 0.37 ;     % 25cm
%     e = abs(a - b) / sqrt(4*a*b) ;
    h = 0.2 ;           % 0.2
%     cBeta = sigmaNormFun(c_prime, epsilon) ;
    dBeta = sigmaNormFun(d_prime, epsilon) ;
    
    Pj = [xj ; yj] ;
    Pk = [xk ; yk] ;
    Pc = [xobs ; yobs] ;
    % Compute closest point between the robot center and the obstacle
    % circumference (ossumming obstacles are circles)
    Pobsj = Pc + (Pj - Pc) * (R /norm(Pj - Pc)) ;
    Pobsk = Pc + (Pk - Pc) * (R /norm(Pk - Pc)) ;
    %Pk = [xobs ; yobs] ;
    
    sigmaNormj = sigmaNormFun(Pobsj - Pj, epsilon) ;
    nij = gradSigmaFun(Pobsj - Pj, epsilon) ;
    
    sigmaNormk = sigmaNormFun(Pobsk - Pk, epsilon) ;
    nik = gradSigmaFun(Pobsk - Pk, epsilon) ;
    
    sigma1j = sigma1Fun(sigmaNormj - dBeta) ;
    sigma1k = sigma1Fun(sigmaNormk - dBeta) ;
    
    phiBetaj = bumpFcn(sigmaNormj/dBeta,h) * (sigma1j - 1) ;
    phiBetak = bumpFcn(sigmaNormk/dBeta,h) * (sigma1k - 1) ;
    
    phiBetaniknei = phiBetaj.* nij + phiBetak.* nik ;
    
end

== matlab function flockingModel/Flocking3/MATLAB Function ==
  data: xi input; yi input; phiAlphanij output; xj input; yj input; xk input; yk input; phiAlphanik output

function [phiAlphanij, phiAlphanik]  = phiAlphaFcn(xi, yi, xj, yj, xk, yk)
    
    % Parameters
    epsilon = 0.1 ;
    a = 1 ;        % 0 < a <= b
    b = 1 ;
    c = 0.6 ;     % 0.6 
    d = 0.3 ;     % 0.3
    e = abs(a - b) / sqrt(4*a*b) ;
    h = 0.2 ;
    cAlpha = sigmaNormFun(c, epsilon) ;
    dAlpha = sigmaNormFun(d, epsilon) ;
    
    Pi = [xi ; yi] ;
    Pj = [xj ; yj] ;
    Pk = [xk ; yk] ;
    
    sigmaNormj = sigmaNormFun(Pj - Pi, epsilon) ;
    nij = gradSigmaFun(Pj - Pi, epsilon) ;
    
    sigmaNormk = sigmaNormFun(Pk - Pi, epsilon) ;
    nik = gradSigmaFun(Pk - Pi, epsilon) ;
    
    sigma1j = sigma1Fun(sigmaNormj - dAlpha + e) ;
    sigma1k = sigma1Fun(sigmaNormk - dAlpha + e) ;
    
    phiAlphaj = 0.5 * bumpFcn(sigmaNormj/cAlpha,h) * ((a+b)*sigma1j + (a-b)) ;
    phiAlphanij = phiAlphaj.* nij ;
    
    phiAlphak = 0.5 * bumpFcn(sigmaNormk/cAlpha,h) * ((a+b)*sigma1k + (a-b)) ;
    phiAlphanik = phiAlphak.* nik ;
    
end

== matlab function flockingModel/Flocking1/MATLAB Function3 ==
  data: xi input; yi input; phiBetanik output; xobs input; yobs input; R input
function phiBetanik = phiBetaFcn(xi, yi, xobs, yobs, R)
    
    % Parameters
    epsilon = 0.1 ;
%     a = 1 ;        % 0 < a <= b
%     b = 1 ;
%     c_prime = 1 ;     % 60cm
    d_prime = 0.37 ;     % 25cm
%     e = abs(a - b) / sqrt(4*a*b) ;
    h = 0.2 ;           % 0.2
%     cBeta = sigmaNormFun(c_prime, epsilon) ;
    dBeta = sigmaNormFun(d_prime, epsilon) ;
    
    Pi = [xi ; yi] ;
    Pc = [xobs ; yobs] ;
    % Compute closest point between the robot center and the obstacle
    % circumference (ossumming obstacles are circles)
    Pk = Pc + (Pi - Pc) * (R /norm(Pi - Pc)) ;
    %Pk = [xobs ; yobs] ;
    
    sigmaNormk = sigmaNormFun(Pk - Pi, epsilon) ;
    nik = gradSigmaFun(Pk - Pi, epsilon) ;
    
    sigma1k = sigma1Fun(sigmaNormk - dBeta) ;
    
    phiBetak = bumpFcn(sigmaNormk/dBeta,h) * (sigma1k - 1) ;
    phiBetanik = phiBetak.* nik ;
    
end

== matlab function flockingModel/Flocking3/MATLAB Function1 ==
  data: phiAlphanij input; phiAlphanij_int input; phiAlphanik input; phiAlphanik_int input; phiBetak input; thetai input; Vi output; omegai output; ui_gamma input; phiBetanei input

function [Vi, omegai]  = ctrlLaw(phiAlphanij, phiAlphanij_int, phiAlphanik, phiAlphanik_int, phiBetak, thetai, ui_gamma, phiBetanei)
    
    % Control gains and parameters
    Kp = 4.5 ;%4.5 ; %5.50 ; % 7.5
    Ki = 0.45 ; %0.35 ; % 0.05
    l = 0.01 ;
    
    cBeta = 0.2; % 0.2
    
    Ktheta = [cos(thetai), sin(thetai) ;
              -sin(thetai)/l, cos(thetai)/l ] ;
    
    hx_dot = Kp * phiAlphanij(1,1) + Ki * phiAlphanij_int(1,1) + Kp * phiAlphanik(1,1) + Ki * phiAlphanik_int(1,1) + cBeta * (phiBetak(1,1) + phiBetanei(1,1)) + ui_gamma(1,1) ;
    hy_dot = Kp * phiAlphanij(2,1) + Ki * phiAlphanij_int(2,1) + Kp * phiAlphanik(2,1) + Ki * phiAlphanik_int(2,1) + cBeta * (phiBetak(2,1) + phiBetanei(2,1)) + ui_gamma(2,1) ;
    
    %hx_dot = Kp * phiAlphanij(1,1) + Ki * phiAlphanij_int(1,1) + Kp * phiAlphanik(1,1) + Ki * phiAlphanik_int(1,1) + cBeta * (phiBetak(1,1)) + ui_gamma(1,1) ;
    %hy_dot = Kp * phiAlphanij(2,1) + Ki * phiAlphanij_int(2,1) + Kp * phiAlphanik(2,1) + Ki * phiAlphanik_int(2,1) + cBeta * (phiBetak(2,1)) + ui_gamma(2,1) ;
    
    Ui = Ktheta * [hx_dot ; hy_dot] ;
    Vi = Ui(1,1) ;
    omegai = Ui(2,1) ;
    
end

== matlab function flockingModel/Flocking3/MATLAB Function2 ==
  data: xi input; yi input; ui_gamma output; xr input; yr input

function ui_gamma   = naviFeedback(xi, yi, xr, yr)
    
    % Control gains
    c_gamma = 0.04 ;
    xmin = -0.03 ;
    xmax = 0.03 ;
    
    Pi = [xi ; yi ] ;
    Pr = [xr ; yr ] ;
    
    ui_gamma = (-1).* satFcn(c_gamma.*(Pi - Pr), xmin, xmax) ;
    
    %Vi_gamma =  - ui_gamma(1,1) ;
    %omegai_gamma = - ui_gamma(2,1) ;
    
end

== matlab function flockingModel/Flocking1/MATLAB Function4 ==
  data: xj input; yj input; xk input; yk input; phiBetaniknei output; xobs input; yobs input; R input
function phiBetaniknei = phiBetaFcn(xj, yj, xk, yk, xobs, yobs, R)
    
    % Parameters
    epsilon = 0.1 ;
%     a = 1 ;        % 0 < a <= b
%     b = 1 ;
%     c_prime = 1 ;     % 60cm
    d_prime = 0.37 ;     % 25cm
%     e = abs(a - b) / sqrt(4*a*b) ;
    h = 0.2 ;           % 0.2
%     cBeta = sigmaNormFun(c_prime, epsilon) ;
    dBeta = sigmaNormFun(d_prime, epsilon) ;
    
    Pj = [xj ; yj] ;
    Pk = [xk ; yk] ;
    Pc = [xobs ; yobs] ;
    % Compute closest point between the robot center and the obstacle
    % circumference (ossumming obstacles are circles)
    Pobsj = Pc + (Pj - Pc) * (R /norm(Pj - Pc)) ;
    Pobsk = Pc + (Pk - Pc) * (R /norm(Pk - Pc)) ;
    %Pk = [xobs ; yobs] ;
    
    sigmaNormj = sigmaNormFun(Pobsj - Pj, epsilon) ;
    nij = gradSigmaFun(Pobsj - Pj, epsilon) ;
    
    sigmaNormk = sigmaNormFun(Pobsk - Pk, epsilon) ;
    nik = gradSigmaFun(Pobsk - Pk, epsilon) ;
    
    sigma1j = sigma1Fun(sigmaNormj - dBeta) ;
    sigma1k = sigma1Fun(sigmaNormk - dBeta) ;
    
    phiBetaj = bumpFcn(sigmaNormj/dBeta,h) * (sigma1j - 1) ;
    phiBetak = bumpFcn(sigmaNormk/dBeta,h) * (sigma1k - 1) ;
    
    phiBetaniknei = phiBetaj.* nij + phiBetak.* nik ;
    
end

== matlab function flockingModel/Flocking3/MATLAB Function3 ==
  data: xi input; yi input; phiBetanik output; xobs input; yobs input; R input
function phiBetanik = phiBetaFcn(xi, yi, xobs, yobs, R)
    
    % Parameters
    epsilon = 0.1 ;
%     a = 1 ;        % 0 < a <= b
%     b = 1 ;
%     c_prime = 1 ;     % 60cm
    d_prime = 0.37 ;     % 25cm
%     e = abs(a - b) / sqrt(4*a*b) ;
    h = 0.2 ;           % 0.2
%     cBeta = sigmaNormFun(c_prime, epsilon) ;
    dBeta = sigmaNormFun(d_prime, epsilon) ;
    
    Pi = [xi ; yi] ;
    Pc = [xobs ; yobs] ;
    % Compute closest point between the robot center and the obstacle
    % circumference (ossumming obstacles are circles)
    Pk = Pc + (Pi - Pc) * (R /norm(Pi - Pc)) ;
    %Pk = [xobs ; yobs] ;
    
    sigmaNormk = sigmaNormFun(Pk - Pi, epsilon) ;
    nik = gradSigmaFun(Pk - Pi, epsilon) ;
    
    sigma1k = sigma1Fun(sigmaNormk - dBeta) ;
    
    phiBetak = bumpFcn(sigmaNormk/dBeta,h) * (sigma1k - 1) ;
    phiBetanik = phiBetak.* nik ;
    
end

== matlab function flockingModel/Flocking3/MATLAB Function4 ==
  data: xj input; yj input; xk input; yk input; phiBetaniknei output; xobs input; yobs input; R input
function phiBetaniknei = phiBetaFcn(xj, yj, xk, yk, xobs, yobs, R)
    
    % Parameters
    epsilon = 0.1 ;
%     a = 1 ;        % 0 < a <= b
%     b = 1 ;
%     c_prime = 1 ;     % 60cm
    d_prime = 0.37 ;     % 25cm
%     e = abs(a - b) / sqrt(4*a*b) ;
    h = 0.2 ;           % 0.2
%     cBeta = sigmaNormFun(c_prime, epsilon) ;
    dBeta = sigmaNormFun(d_prime, epsilon) ;
    
    Pj = [xj ; yj] ;
    Pk = [xk ; yk] ;
    Pc = [xobs ; yobs] ;
    % Compute closest point between the robot center and the obstacle
    % circumference (ossumming obstacles are circles)
    Pobsj = Pc + (Pj - Pc) * (R /norm(Pj - Pc)) ;
    Pobsk = Pc + (Pk - Pc) * (R /norm(Pk - Pc)) ;
    %Pk = [xobs ; yobs] ;
    
    sigmaNormj = sigmaNormFun(Pobsj - Pj, epsilon) ;
    nij = gradSigmaFun(Pobsj - Pj, epsilon) ;
    
    sigmaNormk = sigmaNormFun(Pobsk - Pk, epsilon) ;
    nik = gradSigmaFun(Pobsk - Pk, epsilon) ;
    
    sigma1j = sigma1Fun(sigmaNormj - dBeta) ;
    sigma1k = sigma1Fun(sigmaNormk - dBeta) ;
    
    phiBetaj = bumpFcn(sigmaNormj/dBeta,h) * (sigma1j - 1) ;
    phiBetak = bumpFcn(sigmaNormk/dBeta,h) * (sigma1k - 1) ;
    
    phiBetaniknei = phiBetaj.* nij + phiBetak.* nik ;
    
end
